simulink model "pract6_Simulink"  (R2026a)
settings: Solver=VariableStepAuto  StopTime=0.005  MaxStep=1e-6
settings Model: Creator=elmik  LastModifiedBy=elmik

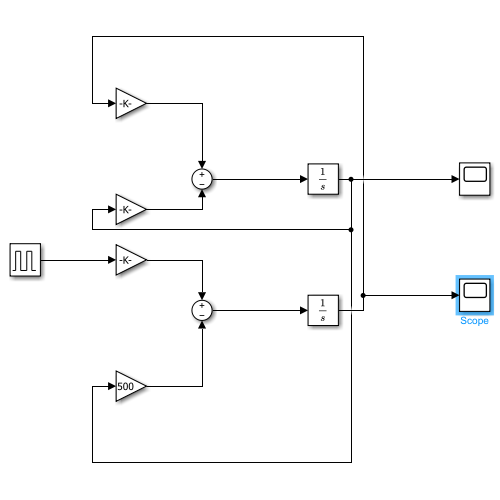
[thumbnail: Simulink's stored preview of the top-level diagram]
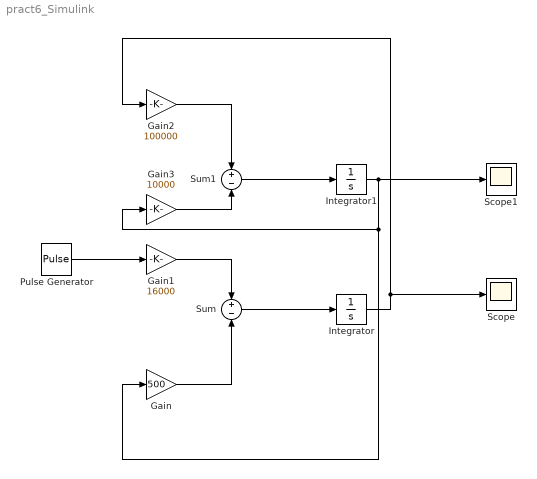
== system pract6_Simulink ==
  Gain : Gain  Gain=500
  Gain1 : Gain  Gain=16000
  Gain2 : Gain  Gain=100000
  Gain3 : Gain  Gain=10000
  Integrator : Integrator
  Integrator1 : Integrator
  Pulse Generator : DiscretePulseGenerator  PulseType=Time based  Period=1e-5  PulseWidth=40
  Scope : Scope
      settings: ActiveDisplayYMinimum=-0.17312047082287454  ActiveDisplayYMaximum=1.5580842374058712
  Scope1 : Scope
      settings: ActiveDisplayYMinimum=-4.1728556513914716  ActiveDisplayYMaximum=37.555700862523253
  Sum : Sum  Inputs=+-
  Sum1 : Sum  Inputs=+-
  wires:
  Sum/1 -> Integrator/1
  Gain/1 -> Sum/2
  Gain1/1 -> Sum/1
  Pulse Generator/1 -> Gain1/1
  Gain2/1 -> Sum1/1
  Gain3/1 -> Sum1/2
  Integrator/1 -> Gain2/1, Scope/1
  Integrator1/1 -> Gain3/1, Gain/1, Scope1/1
  Sum1/1 -> Integrator1/1
